simulink model "supple1a"  (R2022a)
settings: Solver=FixedStepAuto  StartTime=0.0  StopTime=inf  FixedStep=0.1  RelTol=1e-3
(part 2 of 2)

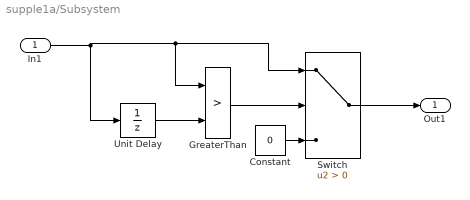
== system supple1a/Subsystem ==
  In1 : Inport
  Constant : Constant  Value=0  OutDataTypeStr=boolean
  GreaterThan : RelationalOperator  Operator=>  OutDataTypeStr=boolean  RndMeth=Simplest  InputSameDT=off
  Switch : Switch  Criteria=u2 > Threshold  SaturateOnIntegerOverflow=off  InputSameDT=off
  Unit Delay : UnitDelay  SampleTime=-1  HasFrameUpgradeWarning=on
  Out1 : Outport
  wires:
  In1/1 -> Unit Delay/1, GreaterThan/1, Switch/1
  Unit Delay/1 -> GreaterThan/2
  GreaterThan/1 -> Switch/2
  Switch/1 -> Out1/1
  Constant/1 -> Switch/3

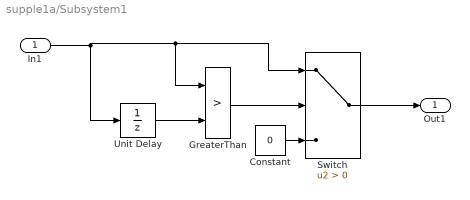
== system supple1a/Subsystem1 ==
  In1 : Inport
  Constant : Constant  Value=0  OutDataTypeStr=boolean
  GreaterThan : RelationalOperator  Operator=>  OutDataTypeStr=boolean  RndMeth=Simplest  InputSameDT=off
  Switch : Switch  Criteria=u2 > Threshold  SaturateOnIntegerOverflow=off  InputSameDT=off
  Unit Delay : UnitDelay  SampleTime=-1  HasFrameUpgradeWarning=on
  Out1 : Outport
  wires:
  In1/1 -> Unit Delay/1, GreaterThan/1, Switch/1
  Unit Delay/1 -> GreaterThan/2
  GreaterThan/1 -> Switch/2
  Switch/1 -> Out1/1
  Constant/1 -> Switch/3

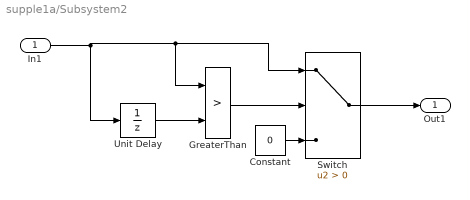
== system supple1a/Subsystem2 ==
  In1 : Inport
  Constant : Constant  Value=0  OutDataTypeStr=boolean
  GreaterThan : RelationalOperator  Operator=>  OutDataTypeStr=boolean  RndMeth=Simplest  InputSameDT=off
  Switch : Switch  Criteria=u2 > Threshold  SaturateOnIntegerOverflow=off  InputSameDT=off
  Unit Delay : UnitDelay  SampleTime=-1  HasFrameUpgradeWarning=on
  Out1 : Outport
  wires:
  In1/1 -> Unit Delay/1, GreaterThan/1, Switch/1
  Unit Delay/1 -> GreaterThan/2
  GreaterThan/1 -> Switch/2
  Switch/1 -> Out1/1
  Constant/1 -> Switch/3

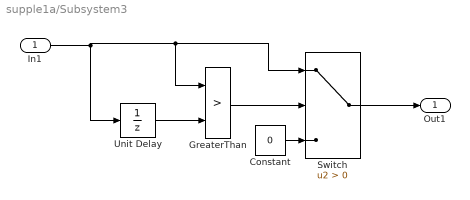
== system supple1a/Subsystem3 ==
  In1 : Inport
  Constant : Constant  Value=0  OutDataTypeStr=boolean
  GreaterThan : RelationalOperator  Operator=>  OutDataTypeStr=boolean  RndMeth=Simplest  InputSameDT=off
  Switch : Switch  Criteria=u2 > Threshold  SaturateOnIntegerOverflow=off  InputSameDT=off
  Unit Delay : UnitDelay  SampleTime=-1  HasFrameUpgradeWarning=on
  Out1 : Outport
  wires:
  In1/1 -> Unit Delay/1, GreaterThan/1, Switch/1
  Unit Delay/1 -> GreaterThan/2
  GreaterThan/1 -> Switch/2
  Switch/1 -> Out1/1
  Constant/1 -> Switch/3

== stateflow chart supple1a/Chart ==
  state DigitalClock
    du:
    ticks= mod(ticks+1, 11);
    state Change_mode
      state Minutes
        en,du:
        Minutes =Changetime(Minutes,60,up,down)
      state Hours
        en,du:
        Hours = Changetime(Hours,24,up,down)
      state Seconds
        en,du:
        Seconds=Changetime(Seconds,60,up,down)
      (default) -> Hours
      Minutes -> Seconds : [m==1]
      Hours -> Minutes : [m==1]
      Seconds -> Hours : [m==1]
    state Normal_mode
      Normal_mode -> (junction 132) [order 1]
      (junction 132) -> (junction 136) [order 1] : [Hours==Alarm_H&Minutes==Alarm_M&Seconds==Alarm_S&SetAlarm]{Alarm=true}
      (junction 132) -> (junction 140) [order 3]
      (junction 132) -> (junction 140) [order 2] : [Alarm==1&m==1]{Alarm=false}
      (junction 136) -> (junction 143)
      (junction 143) -> (junction 140)
    state Alarm
      state Alarm_M
        en,du:
        Alarm_M =Changetime(Alarm_M,60,up,down)
      state Alarm_H
        en,du:
        Alarm_H = Changetime(Alarm_H,24,up,down)
      state Alarm_S
        en,du:
        Alarm_S=Changetime(Alarm_S,60,up,down)
      (default) -> Alarm_H
      Alarm_M -> Alarm_S : [m==1]
      Alarm_H -> Alarm_M : [m==1]
      Alarm_S -> Alarm_H : [m==1]
    DigitalClock -> (junction 180)
    (junction 180) -> (junction 179) [order 1] : [ticks ==10]
        | {Seconds = Seconds +1;
        | ticks = 0;}
    (junction 179) -> (junction 186) [order 1] : [Seconds == 60]
        | {Minutes = Minutes + 1;
        | Seconds = 0;}
    (junction 186) -> (junction 181) [order 1] : [Minutes == 60]
        | {Hours = Hours +1;
        | Minutes =0;}
    (junction 181) -> (junction 183) [order 1] : [Hours == 24]{Hours =0}
    (junction 180) -> (junction 182) [order 2]
    (junction 179) -> (junction 184) [order 2]
    (junction 186) -> (junction 185) [order 2]
    (junction 181) -> (junction 196) [order 2]
    (junction 183) -> (junction 191)
    (junction 184) -> (junction 182)
    (junction 185) -> (junction 184)
    (junction 196) -> (junction 185)
    (junction 191) -> (junction 196)
    Normal_mode -> Change_mode [order 1] : [M == 1]{ChangeTime=true;}
    Change_mode -> Alarm : [M==1]{SetAlarm = true;
        | ChangeTime=false;
        | ChangeAlarm=true;}
    (default) -> Normal_mode
    Alarm -> Normal_mode : [M==1]{ChangeAlarm=false}
  state mod_val = Changetime(init_val,max_val,up1,down1) [function]
    (default) -> (junction 103)
    (junction 103) -> (junction 108) [order 1] : [up1==1]{mod_val=init_val+1;}
    (junction 108) -> (junction 112) [order 1] : [mod_val == max_val]
        | {mod_val=uint8(0);}
    (junction 103) -> (junction 110) [order 3] : {mod_val = init_val}
    (junction 103) -> (junction 110) [order 2] : [down1==1&init_val>0]
        | {mod_val= init_val -1;}
    (junction 108) -> (junction 114) [order 2]
    (junction 112) -> (junction 117)
    (junction 114) -> (junction 110)
    (junction 117) -> (junction 114)
  (default) -> DigitalClock
  data: init_val function_input; max_val function_input; mod_val function_output uint8; up1 function_input; down1 function_input; Hours output uint8 [0..24] =uint8(0); Minutes output uint8 [0..60] =uint8(0); Seconds output uint8 [0..60] =uint8(0); M input boolean; m input boolean; up input boolean; down input boolean; ticks local uint8 [0..10] =uint8(0); Alarm output boolean =false; Alarm_H output =uint8(0); Alarm_M output =uint8(0); Alarm_S output =uint8(0); SetAlarm local boolean =false; ChangeTime output boolean =false; ChangeAlarm output boolean =false
